simulink model "Dyn_PointMass_r2019b"  (R2022b)
settings: Solver=ode4  StartTime=0.0  StopTime=simInit.TSIM  FixedStep=simInit.dt  MaxStep=simInit.dt  RelTol=1e-3
InitFcn:
  | close all
undefined symbols (not defined in the file): constr, DE2019, DiscIntNeverNeededParam, ENVMT, params, simInit
libraries: simulink x15, simulink_extras x2
(part 1 of 2)
Description:
  | % Copyright 2020 Delft University of Technology
  | %
  | % Licensed under the Apache License, Version 2.0 (the "License");
  | % you may not use this file except in compliance with the License.
  | % You may obtain a copy of the License at
  | %
  | %      http://www.apache.org/licenses/LICENSE-2.0
  | %
  | % Unless required by applicable law or agreed to in writing, software
  | % distributed under the License is distributed on an "AS IS" BASIS,
  | % WITHOUT WARRANTIES OR CONDITIONS OF ANY KIND, either express or implied.
  | % See the License for the specific language governing permissions and
  | % limitations under the License.
settings Model: SimulationMode=accelerator  NumberOfSteps=50  ExtModeTrigDuration=100  Creator=Sebastian  LastModifiedBy=jesse
settings SolverCC: SolverJacobianMethodControl=FullAnalytical  AlgebraicLoopSolver=TrustRegion
settings DataIOCC: InitialState=testPoint  SaveFormat=Structure  SignalLogging=off  DSMLogging=off  SaveTime=off  ReturnWorkspaceOutputs=off  StateSaveName=tmp_raccel_xout  SignalLoggingName=logged_signals  LoggingFileName=log
settings OptimizationCC: BlockReduction=off  EfficientMapNaN2IntZero=off  LifeSpan=inf
settings DebuggingCC: ArtificialAlgebraicLoopMsg=none  SaveWithDisabledLinksMsg=none  SaveWithParameterizedLinksMsg=none  MaskedZcDiagnostic=none  IgnoredZcDiagnostic=none  InheritedTsInSrcMsg=none  TasksWithSamePriorityMsg=none  SigSpecEnsureSampleTimeMsg=none  ParameterPrecisionLossMsg=none  BusObjectLabelMismatch=none  RootOutportRequireBusObject=none  UnknownTsInhSupMsg=none  ModelReferenceDataLoggingMessage=none  ModelReferenceSymbolNameMessage=none  InitInArrayFormatMsg=none  SFUnusedDataAndEventsDiag=none  SFUnexpectedBacktrackingDiag=none  SFInvalidInputDataAccessInChartInitDiag=none  SFNoUnconditionalDefaultTransitionDiag=none  SFTransitionOutsideNaturalParentDiag=none  SFUnreachableExecutionPathDiag=none  SFUndirectedBroadcastEventsDiag=none  SFTransitionActionBeforeConditionDiag=none  SFTemporalDelaySmallerThanSampleTimeDiag=none  SFSelfTransitionDiag=none  SFExecutionAtInitializationDiag=none  SFMachineParentedDataDiag=none  UnitsInconsistencyMsg=none  ArithmeticOperatorsInVariantConditions=warning
settings HardwareCC: ProdBitPerLong=64  ProdLongLongMode=on  ProdHWDeviceType=Custom Processor->Custom Processor  TargetBitPerPointer=64  TargetBitPerSizeT=64  TargetBitPerPtrDiffT=64  TargetLargestAtomicFloat=Float  TargetLongLongMode=on  TargetIntDivRoundTo=Zero  TargetEndianess=LittleEndian  TargetWordSize=64  TargetHWDeviceType=Custom Processor->MATLAB Host Computer
settings ModelReferenceCC: EnableRefExpFcnMdlSchedulingChecks=on  PropagateSignalLabelsOutOfModel=off
settings SFSimCC: SimUseLocalCustomCode=off  CustomCodeUndefinedFunction=UseInterfaceOnly
settings CodeAppCC: MaxIdLength=128
settings GRTTargetCC: TargetLangStandard=C89/C90 (ANSI)  CombineOutputUpdateFcns=off  GRTInterface=on
settings ConfigComp: CovMetricSettings=dw  CovSaveCumulativeToWorkspaceVar=on  CovSaveSingleToWorkspaceVar=on  CovExternalEMLEnable=off
settings SimscapeCC: SimscapeNormalizeSystem=off
settings ConfigurationSet: Description=SimMechanics 2G

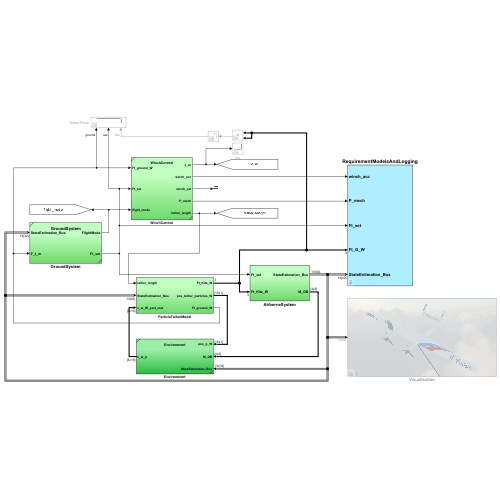
[thumbnail: Simulink's stored preview of the top-level diagram]
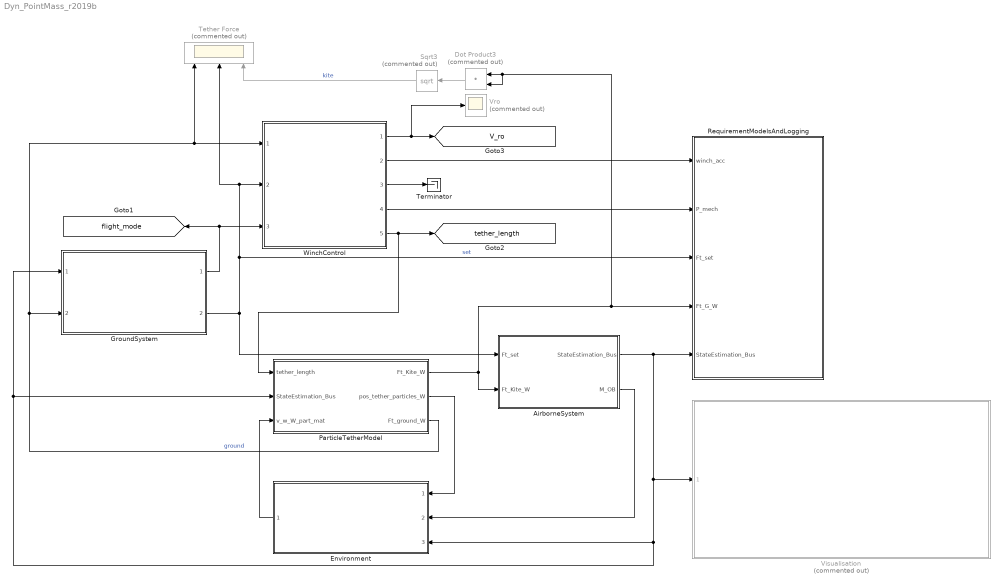
== system Dyn_PointMass_r2019b ==
  AirborneSystem : Subsystem
  Dot Product3 : DotProduct  Commented=on  OutDataTypeStr=Inherit: Inherit via internal rule
  Environment : Subsystem  ReferencedSubsystem=Environment
  GroundSystem : Subsystem  ReferencedSubsystem=GroundSystem
  ParticleTetherModel : Subsystem
  RequirementModelsAndLogging : Subsystem  mask{log_sample_time=0.2}
  Sqrt3 : Sqrt  Commented=on
  Terminator : Terminator
  Tether Force : Scope  Commented=on  NumInputPorts=3
  Visualisation : Subsystem  Commented=on  ReferencedSubsystem=Visualisation  sample_time_vis=1
  Vro : Scope  Commented=on
  WinchControl : Subsystem  ReferencedSubsystem=WinchControl
  tag scope: V_ro=global, flight_mode=global, tether_length=global
  wires:
  GroundSystem/1 -> [flight_mode], WinchControl/3
  GroundSystem/2 -> AirborneSystem/1(Ft_set), RequirementModelsAndLogging/3(Ft_set), Tether Force/2, WinchControl/2  "set"
  AirborneSystem/2(M_OB) -> Environment/2
  AirborneSystem/1(StateEstimation_Bus) -> RequirementModelsAndLogging/5(StateEstimation_Bus), Visualisation/1, GroundSystem/1, ParticleTetherModel/2(StateEstimation_Bus), Environment/3
  ParticleTetherModel/2(pos_tether_particles_W) -> Environment/1
  Environment/1 -> ParticleTetherModel/3(v_w_W_part_mat)
  WinchControl/1 -> Vro/1, [V_ro]
  ParticleTetherModel/3(Ft_ground_W) -> WinchControl/1, Tether Force/1, GroundSystem/2  "ground"
  WinchControl/3 -> Terminator/1
  WinchControl/2 -> RequirementModelsAndLogging/1(winch_acc)
  WinchControl/4 -> RequirementModelsAndLogging/2(P_mech)
  WinchControl/5 -> [tether_length], ParticleTetherModel/1(tether_length)
  Sqrt3/1 -> Tether Force/3  "kite"
  Dot Product3/1 -> Sqrt3/1
  ParticleTetherModel/1(Ft_Kite_W) -> Dot Product3/2, Dot Product3/1, RequirementModelsAndLogging/4(Ft_G_W), AirborneSystem/2(Ft_Kite_W)

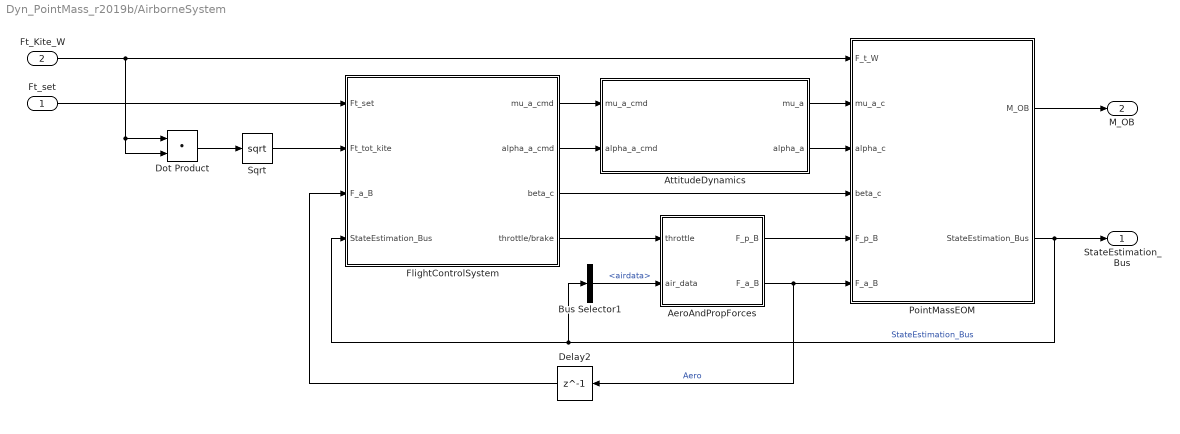
== system Dyn_PointMass_r2019b/AirborneSystem ==
  Ft_set : Inport
  Ft_Kite_W : Inport  Port=2
  AeroAndPropForces : Subsystem
  AttitudeDynamics : Subsystem
  Bus Selector1 : BusSelector  OutputSignals=airdata
  Delay2 : Delay  DelayLength=1  InitialCondition=[0;0;DE2019.mass*ENVMT.g]
  Dot Product : DotProduct  OutDataTypeStr=Inherit: Inherit via internal rule
  FlightControlSystem : Subsystem
  PointMassEOM : Subsystem
  Sqrt : Sqrt
  StateEstimation_Bus : Outport  VectorParamsAs1DForOutWhenUnconnected=off
  M_OB : Outport  Port=2  VectorParamsAs1DForOutWhenUnconnected=off
  wires:
  PointMassEOM/2(StateEstimation_Bus) -> FlightControlSystem/4(StateEstimation_Bus), Bus Selector1/1, StateEstimation_Bus/1  "StateEstimation_Bus"
  PointMassEOM/1(M_OB) -> M_OB/1
  Ft_Kite_W/1 -> PointMassEOM/1(F_t_W), Dot Product/2, Dot Product/1
  Dot Product/1 -> Sqrt/1
  Ft_set/1 -> FlightControlSystem/1(Ft_set)
  Sqrt/1 -> FlightControlSystem/2(Ft_tot_kite)
  FlightControlSystem/4(throttle/brake) -> AeroAndPropForces/1(throttle)
  AeroAndPropForces/1(F_p_B) -> PointMassEOM/5(F_p_B)
  Bus Selector1/1 -> AeroAndPropForces/2(air_data)  "<airdata>"
  AeroAndPropForces/2(F_a_B) -> Delay2/1, PointMassEOM/6(F_a_B)  "Aero"
  AttitudeDynamics/1(mu_a) -> PointMassEOM/2(mu_a_c)
  AttitudeDynamics/2(alpha_a) -> PointMassEOM/3(alpha_c)
  FlightControlSystem/1(mu_a_cmd) -> AttitudeDynamics/1(mu_a_cmd)
  FlightControlSystem/2(alpha_a_cmd) -> AttitudeDynamics/2(alpha_a_cmd)
  FlightControlSystem/3(beta_c) -> PointMassEOM/4(beta_c)
  Delay2/1 -> FlightControlSystem/3(F_a_B)

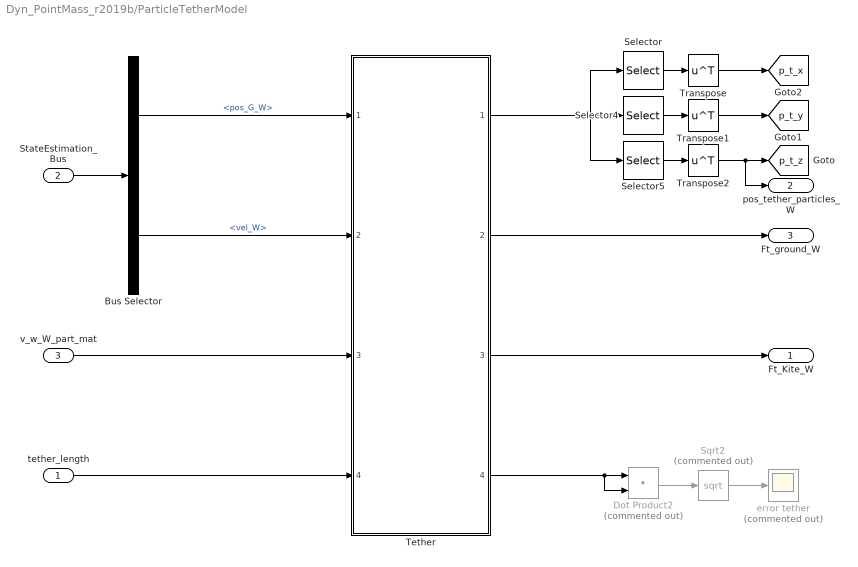
== system Dyn_PointMass_r2019b/ParticleTetherModel ==
  tether_length : Inport
  StateEstimation_Bus : Inport  Port=2
  v_w_W_part_mat : Inport  Port=3
  Bus Selector : BusSelector  OutputSignals=pos_G_W,vel_W
  Dot Product2 : DotProduct  Commented=on  OutDataTypeStr=Inherit: Inherit via internal rule
  Selector : Selector  NumberOfDimensions=2  InputPortWidth=3  IndexOptions=Index vector (dialog),Select all  Indices=1,1  OutputSizes=1,1
  Selector4 : Selector  NumberOfDimensions=2  InputPortWidth=3  IndexOptions=Index vector (dialog),Select all  Indices=2,1  OutputSizes=1,1
  Selector5 : Selector  NumberOfDimensions=2  InputPortWidth=3  IndexOptions=Index vector (dialog),Select all  Indices=3,1  OutputSizes=1,1
  Sqrt2 : Sqrt  Commented=on
  Tether : Subsystem  ReferencedSubsystem=Tether_dynamics_R2019B
  Transpose : Math  Operator=transpose
  Transpose1 : Math  Operator=transpose
  Transpose2 : Math  Operator=transpose
  error tether : Scope  Commented=on
  Ft_Kite_W : Outport  VectorParamsAs1DForOutWhenUnconnected=off
  pos_tether_particles_W : Outport  Port=2  VectorParamsAs1DForOutWhenUnconnected=off
  Ft_ground_W : Outport  Port=3  VectorParamsAs1DForOutWhenUnconnected=off
  tag scope: p_t_x=global, p_t_y=global, p_t_z=global
  wires:
  v_w_W_part_mat/1 -> Tether/3
  StateEstimation_Bus/1 -> Bus Selector/1
  Bus Selector/1 -> Tether/1  "<pos_G_W>"
  Bus Selector/2 -> Tether/2  "<vel_W>"
  Selector4/1 -> Transpose1/1
  Selector5/1 -> Transpose2/1
  Selector/1 -> Transpose/1
  Transpose/1 -> [p_t_x]
  Transpose1/1 -> [p_t_y]
  Transpose2/1 -> pos_tether_particles_W/1, [p_t_z]
  Tether/4 -> Dot Product2/2, Dot Product2/1
  Tether/1 -> Selector/1, Selector5/1, Selector4/1
  Dot Product2/1 -> Sqrt2/1
  Sqrt2/1 -> error tether/1
  Tether/2 -> Ft_ground_W/1
  Tether/3 -> Ft_Kite_W/1
  tether_length/1 -> Tether/4

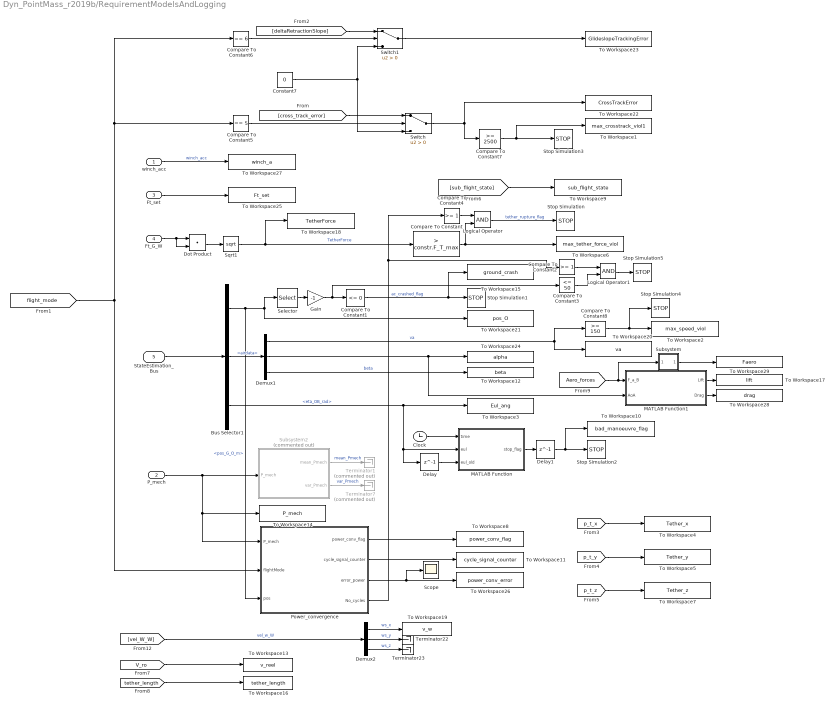
== system Dyn_PointMass_r2019b/RequirementModelsAndLogging ==
  winch_acc : Inport
  P_mech : Inport  Port=2
  Ft_set : Inport  Port=3
  Ft_G_W : Inport  Port=4
  StateEstimation_Bus : Inport  Port=5
  Bus Selector1 : BusSelector  OutputSignals=pos_G_O_m,airdata,eta_OB_rad
  Clock : Clock
  Compare To Constant : simulink/Logic and Bit Operations/Compare To Constant  relop=>  const=constr.F_T_max  OutDataTypeStr=boolean
  Compare To Constant1 : simulink/Logic and Bit Operations/Compare To Constant  relop=<=  const=0  OutDataTypeStr=boolean
  Compare To Constant2 : simulink/Logic and Bit Operations/Compare To Constant  relop=>=  const=1  OutDataTypeStr=boolean
  Compare To Constant3 : simulink/Logic and Bit Operations/Compare To Constant  relop=<=  const=50  OutDataTypeStr=boolean
  Compare To Constant4 : simulink/Logic and Bit Operations/Compare To Constant  relop=>=  const=1  OutDataTypeStr=boolean
  Compare To Constant5 : simulink/Logic and Bit Operations/Compare To Constant  relop===  const=5  OutDataTypeStr=boolean
  Compare To Constant6 : simulink/Logic and Bit Operations/Compare To Constant  relop===  const=6  OutDataTypeStr=boolean
  Compare To Constant7 : simulink/Logic and Bit Operations/Compare To Constant  relop=>=  const=2500  OutDataTypeStr=boolean
  Compare To Constant8 : simulink/Logic and Bit Operations/Compare To Constant  relop=>=  const=150  OutDataTypeStr=boolean
  Constant7 : Constant  Value=0
  Delay : Delay  DelayLength=1  InitialCondition=zeros(3,1)
  Delay1 : Delay  DelayLength=1
  Demux1 : Demux  Outputs=3
  Demux2 : Demux  Outputs=3
  Dot Product : DotProduct  OutDataTypeStr=Inherit: Inherit via internal rule
  Gain : Gain  Gain=-1
  Logical Operator : Logic  AllPortsSameDT=off  OutDataTypeStr=boolean
  Logical Operator1 : Logic  AllPortsSameDT=off  OutDataTypeStr=boolean
  MATLAB Function : MATLAB Function  TreatAsAtomicUnit=on
  MATLAB Function1 : MATLAB Function  TreatAsAtomicUnit=on
  Power_convergence : Subsystem  mask{sample_time=simInit.Ts_power_conv_check, threshold=130000, min_cycles=3, pos_threshold=400}
      mask prompts: threshold "start_threshold"; min_cycles "minimum_cycles"; pos_threshold "maximum position distance"
  Scope : Scope
  Selector : Selector  InputPortWidth=3  IndexOptions=Index vector (dialog)  Indices=3  OutputSizes=1
  Sqrt1 : Sqrt
  Stop Simulation{,1..5} (6 alike) : Stop
  Subsystem : Subsystem
      mask Display: disp('norm()')
  Subsystem2 : Subsystem  Commented=on
  Switch : Switch  Criteria=u2 > Threshold  SaturateOnIntegerOverflow=off  InputSameDT=off
  Switch1 : Switch  Criteria=u2 > Threshold  SaturateOnIntegerOverflow=off  InputSameDT=off
  Terminator1 : Terminator  Commented=on
  Terminator22 : Terminator
  Terminator23 : Terminator
  Terminator7 : Terminator  Commented=on
  To Workspace1 : ToWorkspace  VariableName=max_crosstrack_viol1  SampleTime=-1
      settings: MaxDataPoints=1
  To Workspace10 : ToWorkspace  VariableName=bad_manoeuvre_flag  SampleTime=-1
      settings: MaxDataPoints=1
  To Workspace11 : ToWorkspace  VariableName=cycle_signal_counter  SaveFormat=Timeseries  SampleTime=-1
      settings: MaxDataPoints=1  Save2DSignal=2-D array (concatenate along first dimension)
  To Workspace12 : ToWorkspace  VariableName=beta  SaveFormat=Timeseries  SampleTime=simInit.AttLoggingTs
      settings: Save2DSignal=2-D array (concatenate along first dimension)
  To Workspace13 : ToWorkspace  VariableName=v_reel  SaveFormat=Timeseries  SampleTime=simInit.PLoggingTs
  To Workspace14 : ToWorkspace  VariableName=P_mech  SaveFormat=Timeseries  SampleTime=simInit.PLoggingTs
  To Workspace15 : ToWorkspace  VariableName=ground_crash  SampleTime=-1
      settings: MaxDataPoints=1
  To Workspace16 : ToWorkspace  VariableName=tether_length  SaveFormat=Timeseries  SampleTime=simInit.AttLoggingTs
  To Workspace17 : ToWorkspace  VariableName=lift  SaveFormat=Timeseries  SampleTime=simInit.AttLoggingTs
      settings: Save2DSignal=2-D array (concatenate along first dimension)
  To Workspace18 : ToWorkspace  VariableName=TetherForce  SaveFormat=Timeseries  SampleTime=simInit.FtLoggingTs
  To Workspace19 : ToWorkspace  VariableName=v_w  SaveFormat=Timeseries  SampleTime=simInit.PLoggingTs
  To Workspace2 : ToWorkspace  VariableName=max_speed_viol  SampleTime=-1
      settings: MaxDataPoints=1
  To Workspace20 : ToWorkspace  VariableName=va  SaveFormat=Timeseries  SampleTime=simInit.AttLoggingTs
      settings: Save2DSignal=2-D array (concatenate along first dimension)
  To Workspace21 : ToWorkspace  VariableName=pos_O  SaveFormat=Timeseries  SampleTime=simInit.PLoggingTs
      settings: Save2DSignal=2-D array (concatenate along first dimension)
  To Workspace22 : ToWorkspace  VariableName=CrossTrackError  SaveFormat=Timeseries  SampleTime=simInit.CteLoggingTs
      settings: Save2DSignal=2-D array (concatenate along first dimension)
  To Workspace23 : ToWorkspace  VariableName=GlideslopeTrackingError  SaveFormat=Timeseries  SampleTime=simInit.GSLoggingTs
      settings: Save2DSignal=2-D array (concatenate along first dimension)
  To Workspace24 : ToWorkspace  VariableName=alpha  SaveFormat=Timeseries  SampleTime=simInit.AttLoggingTs
      settings: Save2DSignal=2-D array (concatenate along first dimension)
  To Workspace25 : ToWorkspace  VariableName=Ft_set  SaveFormat=Timeseries  SampleTime=simInit.FtLoggingTs
  To Workspace26 : ToWorkspace  VariableName=power_conv_error  SaveFormat=Timeseries  SampleTime=-1
      settings: Save2DSignal=2-D array (concatenate along first dimension)
  To Workspace27 : ToWorkspace  VariableName=winch_a  SaveFormat=Timeseries  SampleTime=simInit.PLoggingTs
  To Workspace28 : ToWorkspace  VariableName=drag  SaveFormat=Timeseries  SampleTime=simInit.AttLoggingTs
      settings: Save2DSignal=2-D array (concatenate along first dimension)
  To Workspace29 : ToWorkspace  VariableName=Faero  SaveFormat=Timeseries  SampleTime=simInit.AttLoggingTs
      settings: Save2DSignal=2-D array (concatenate along first dimension)
  To Workspace3 : ToWorkspace  VariableName=Eul_ang  SaveFormat=Timeseries  SampleTime=simInit.PLoggingTs
      settings: Save2DSignal=2-D array (concatenate along first dimension)
  To Workspace4 : ToWorkspace  VariableName=Tether_x  SaveFormat=Timeseries  SampleTime=simInit.PLoggingTs
      settings: Save2DSignal=2-D array (concatenate along first dimension)
  To Workspace5 : ToWorkspace  VariableName=Tether_y  SaveFormat=Timeseries  SampleTime=simInit.PLoggingTs
      settings: Save2DSignal=2-D array (concatenate along first dimension)
  To Workspace6 : ToWorkspace  VariableName=max_tether_force_viol  SampleTime=-1
      settings: MaxDataPoints=1
  To Workspace7 : ToWorkspace  VariableName=Tether_z  SaveFormat=Timeseries  SampleTime=simInit.PLoggingTs
      settings: Save2DSignal=2-D array (concatenate along first dimension)
  To Workspace8 : ToWorkspace  VariableName=power_conv_flag  SampleTime=-1
      settings: MaxDataPoints=1
  To Workspace9 : ToWorkspace  VariableName=sub_flight_state  SaveFormat=Timeseries  SampleTime=simInit.FtLoggingTs
  wires:
  Bus Selector1/1 -> Power_convergence/3(pos), Selector/1, To Workspace21/1  "<pos_G_O_m>"
  Gain/1 -> Compare To Constant3/1, Compare To Constant1/1
  Compare To Constant1/1 -> To Workspace15/1, Stop Simulation1/1  "ac_crashed_flag"
  Selector/1 -> Gain/1
  winch_acc/1 -> To Workspace27/1  "winch_acc"
  Logical Operator/1 -> Stop Simulation/1  "tether_rupture_flag"
  Sqrt1/1 -> To Workspace18/1, Compare To Constant/1  "TetherForce"
  StateEstimation_Bus/1 -> Bus Selector1/1
  Power_convergence/1(power_conv_flag) -> To Workspace8/1
  Power_convergence/2(cycle_signal_counter) -> To Workspace11/1
  [vel_W_W] -> Demux2/1  "vel_w_W"
  Bus Selector1/2 -> Demux1/1  "<airdata>"
  Switch/1 -> To Workspace22/1, Compare To Constant7/1
  Subsystem2/1(mean_Pmech) -> Terminator1/1  "mean_Pmech"
  Subsystem2/2(var_Pmech) -> Terminator7/1  "var_Pmech"
  Demux1/1 -> To Workspace20/1, Compare To Constant8/1  "va"
  Demux1/3 -> To Workspace12/1  "beta"
  Demux2/3 -> Terminator23/1  "ws_z"
  Demux2/2 -> Terminator22/1  "ws_y"
  Demux2/1 -> To Workspace19/1  "ws_x"
  Ft_G_W/1 -> Dot Product/2, Dot Product/1
  Dot Product/1 -> Sqrt1/1
  Clock/1 -> MATLAB Function/1(time)
  Compare To Constant4/1 -> Logical Operator/1
  Compare To Constant/1 -> Logical Operator/2, To Workspace6/1
  [flight_mode] -> Compare To Constant6/1, Compare To Constant5/1, Power_convergence/2(flightMode)
  P_mech/1 -> Power_convergence/1(P_mech), To Workspace14/1, Subsystem2/1(P_mech)
  Compare To Constant5/1 -> Switch/2
  [cross_track_error] -> Switch/1
  Switch1/1 -> To Workspace23/1
  [deltaRetractionSlope] -> Switch1/1
  Compare To Constant6/1 -> Switch1/2
  Constant7/1 -> Switch1/3, Switch/3
  Ft_set/1 -> To Workspace25/1
  Power_convergence/3(error_power) -> Scope/1, To Workspace26/1
  Compare To Constant7/1 -> Stop Simulation3/1, To Workspace1/1
  Compare To Constant8/1 -> To Workspace2/1, Stop Simulation4/1
  Bus Selector1/3 -> Delay/1, MATLAB Function/2(eul), To Workspace3/1  "<eta_OB_rad>"
  [p_t_y] -> To Workspace5/1
  [p_t_x] -> To Workspace4/1
  [p_t_z] -> To Workspace7/1
  [sub_flight_state] -> To Workspace9/1
  Delay/1 -> MATLAB Function/3(eul_old)
  MATLAB Function/1(stop_flag) -> Delay1/1
  Delay1/1 -> Stop Simulation2/1, To Workspace10/1
  [V_ro] -> To Workspace13/1
  [tether_length] -> To Workspace16/1
  Power_convergence/4(No_cycles) -> Compare To Constant2/1, Compare To Constant4/1
  Compare To Constant2/1 -> Logical Operator1/1
  Compare To Constant3/1 -> Logical Operator1/2
  Logical Operator1/1 -> Stop Simulation5/1
  MATLAB Function1/1(Lift) -> To Workspace17/1
  [Aero_forces] -> Subsystem/1(In1), MATLAB Function1/1(F_a_B)
  MATLAB Function1/2(Drag) -> To Workspace28/1
  Demux1/2 -> MATLAB Function1/2(AoA), To Workspace24/1
  Subsystem/1(Out1) -> To Workspace29/1

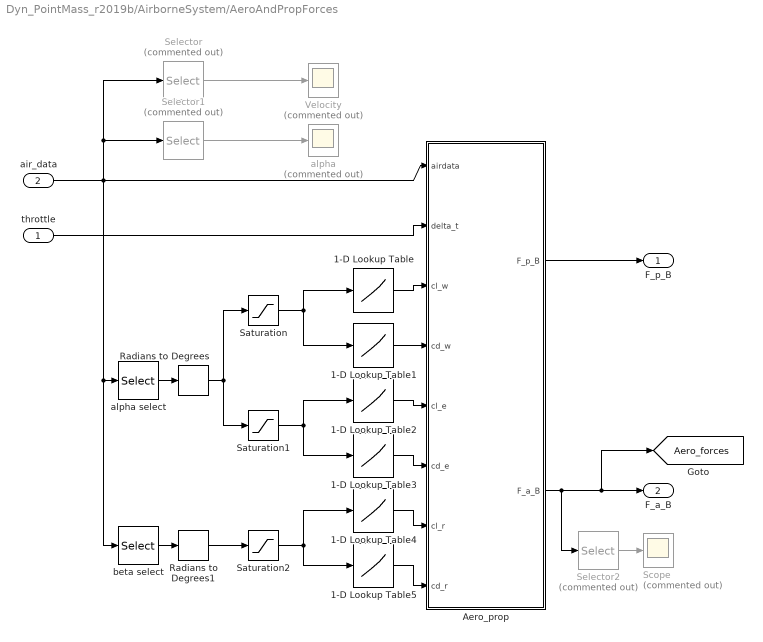
== system Dyn_PointMass_r2019b/AirborneSystem/AeroAndPropForces ==
  throttle : Inport
  air_data : Inport  Port=2
  1-D Lookup Table : Lookup_n-D  NumberOfTableDimensions=1  BreakpointsForDimension1=DE2019.initAircraft.alpha  BreakpointsForDimension2=[1 1]  Table=DE2019.initAircraft.wing_cL_Static'  InternalRulePriority=Speed  RndMeth=Simplest
  1-D Lookup Table1 : Lookup_n-D  NumberOfTableDimensions=1  BreakpointsForDimension1=DE2019.initAircraft.alpha  BreakpointsForDimension2=[1 1]  Table=DE2019.initAircraft.wing_cD_Static'  InternalRulePriority=Speed  RndMeth=Simplest
  1-D Lookup Table2 : Lookup_n-D  NumberOfTableDimensions=1  BreakpointsForDimension1=DE2019.alpha  BreakpointsForDimension2=[1 1]  Table=DE2019.el_cL'  InternalRulePriority=Speed  RndMeth=Simplest
  1-D Lookup Table3 : Lookup_n-D  NumberOfTableDimensions=1  BreakpointsForDimension1=DE2019.alpha  BreakpointsForDimension2=[1 1]  Table=DE2019.el_cD'  InternalRulePriority=Speed  RndMeth=Simplest
  1-D Lookup Table4 : Lookup_n-D  NumberOfTableDimensions=1  BreakpointsForDimension1=DE2019.alpha  BreakpointsForDimension2=[1 1]  Table=DE2019.vs_cL'  InternalRulePriority=Speed  RndMeth=Simplest
  1-D Lookup Table5 : Lookup_n-D  NumberOfTableDimensions=1  BreakpointsForDimension1=DE2019.alpha  BreakpointsForDimension2=[1 1]  Table=DE2019.vs_cD'  InternalRulePriority=Speed  RndMeth=Simplest
  Aero_prop : MATLAB Function  TreatAsAtomicUnit=on
  Radians to Degrees : simulink_extras/Transformations/Radians to Degrees
  Radians to Degrees1 : simulink_extras/Transformations/Radians to Degrees
  Saturation : Saturate  UpperLimit=max(DE2019.initAircraft.alpha)  LowerLimit=min(DE2019.initAircraft.alpha)
  Saturation1 : Saturate  UpperLimit=max(DE2019.alpha)  LowerLimit=min(DE2019.alpha)
  Saturation2 : Saturate  UpperLimit=max(DE2019.alpha)  LowerLimit=min(DE2019.alpha)
  Scope : Scope  Commented=on
  Selector : Selector  Commented=on  InputPortWidth=3  IndexOptions=Index vector (dialog)  Indices=[1]  OutputSizes=1
  Selector1 : Selector  Commented=on  InputPortWidth=3  IndexOptions=Index vector (dialog)  Indices=2  OutputSizes=1
  Selector2 : Selector  Commented=on  InputPortWidth=3  IndexOptions=Index vector (dialog)  Indices=3  OutputSizes=1
  Velocity : Scope  Commented=on
  alpha : Scope  Commented=on
  alpha select : Selector  InputPortWidth=3  IndexOptions=Index vector (dialog)  Indices=2  OutputSizes=1
  beta select : Selector  InputPortWidth=3  IndexOptions=Index vector (dialog)  Indices=3  OutputSizes=1
  F_p_B : Outport  VectorParamsAs1DForOutWhenUnconnected=off
  F_a_B : Outport  Port=2  VectorParamsAs1DForOutWhenUnconnected=off
  tag scope: Aero_forces=global
  wires:
  Aero_prop/1(F_p_B) -> F_p_B/1
  throttle/1 -> Aero_prop/2(delta_t)
  Selector/1 -> Velocity/1
  Selector1/1 -> alpha/1
  1-D Lookup Table/1 -> Aero_prop/3(cl_w)
  1-D Lookup Table1/1 -> Aero_prop/4(cd_w)
  Saturation/1 -> 1-D Lookup Table/1, 1-D Lookup Table1/1
  Saturation1/1 -> 1-D Lookup Table3/1, 1-D Lookup Table2/1
  alpha select/1 -> Radians to Degrees/1
  Radians to Degrees/1 -> Saturation1/1, Saturation/1
  1-D Lookup Table2/1 -> Aero_prop/5(cl_e)
  1-D Lookup Table3/1 -> Aero_prop/6(cd_e)
  1-D Lookup Table4/1 -> Aero_prop/7(cl_r)
  1-D Lookup Table5/1 -> Aero_prop/8(cd_r)
  beta select/1 -> Radians to Degrees1/1
  Radians to Degrees1/1 -> Saturation2/1
  Saturation2/1 -> 1-D Lookup Table4/1, 1-D Lookup Table5/1
  Selector2/1 -> Scope/1
  Aero_prop/2(F_a_B) -> [Aero_forces], F_a_B/1, Selector2/1
  air_data/1 -> Selector/1, Selector1/1, Aero_prop/1(airdata), beta select/1, alpha select/1

== system Dyn_PointMass_r2019b/AirborneSystem/AttitudeDynamics ==
  mu_a_cmd : Inport
  alpha_a_cmd : Inport  Port=2
  Scope : Scope  Commented=on  NumInputPorts=2
  SecondOrderReferenceModel_alpha_a : Subsystem  mask{omega0_max=params.w0_alpha, zeta0=1, y_max=constr.alpha_a_max, y_min=constr.alpha_a_min, yd_max=inf, yd_min=-inf, y2d_max=inf, y2d_min=-inf}
  SecondOrderReferenceModel_mu_a : Subsystem  mask{omega0_max=params.w0_mu, zeta0=1, y_max=constr.mu_a_max, y_min=-constr.mu_a_max, yd_max=inf, yd_min=-inf, y2d_max=inf, y2d_min=-inf}
  mu_a : Outport  VectorParamsAs1DForOutWhenUnconnected=off
  alpha_a : Outport  Port=2  VectorParamsAs1DForOutWhenUnconnected=off
  wires:
  mu_a_cmd/1 -> SecondOrderReferenceModel_mu_a/1(y_cmd)
  SecondOrderReferenceModel_alpha_a/1(y_ref) -> Scope/1, alpha_a/1  "alpha_a"
  alpha_a_cmd/1 -> SecondOrderReferenceModel_alpha_a/1(y_cmd), Scope/2
  SecondOrderReferenceModel_mu_a/1(y_ref) -> mu_a/1  "mu_a"

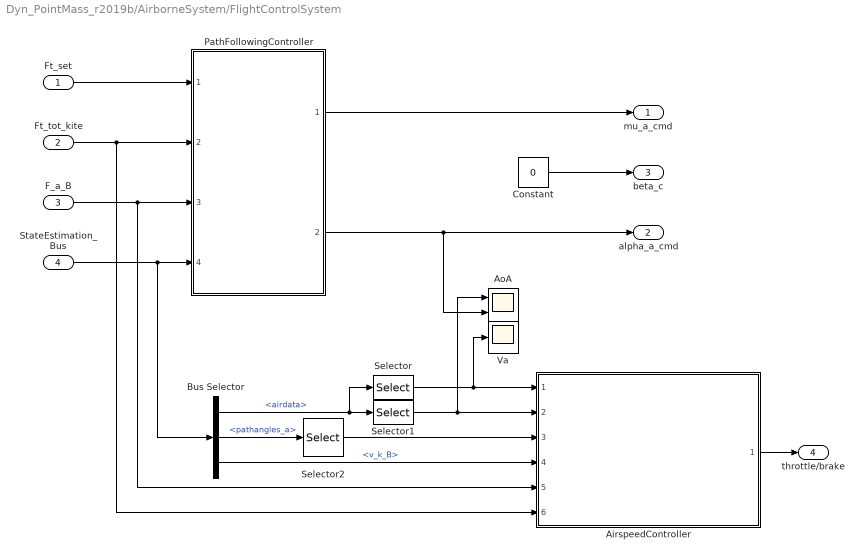
== system Dyn_PointMass_r2019b/AirborneSystem/FlightControlSystem ==
  Ft_set : Inport
  Ft_tot_kite : Inport  Port=2
  F_a_B : Inport  Port=3
  StateEstimation_Bus : Inport  Port=4
  AirspeedController : Subsystem  ReferencedSubsystem=AirspeedController
  AoA : Scope  NumInputPorts=2
  Bus Selector : BusSelector  OutputSignals=airdata,pathangles_a,v_k_B
  Constant : Constant  Value=0
  PathFollowingController : Subsystem  ReferencedSubsystem=PathFollowingController
  Selector : Selector  InputPortWidth=3  IndexOptions=Index vector (dialog)  Indices=1  OutputSizes=1
  Selector1 : Selector  InputPortWidth=3  IndexOptions=Index vector (dialog)  Indices=2  OutputSizes=1
  Selector2 : Selector  InputPortWidth=2  IndexOptions=Index vector (dialog)  Indices=2  OutputSizes=1
  Va : Scope
  mu_a_cmd : Outport  VectorParamsAs1DForOutWhenUnconnected=off
  alpha_a_cmd : Outport  Port=2  VectorParamsAs1DForOutWhenUnconnected=off
  beta_c : Outport  Port=3  VectorParamsAs1DForOutWhenUnconnected=off
  throttle/brake : Outport  Port=4  VectorParamsAs1DForOutWhenUnconnected=off
  wires:
  StateEstimation_Bus/1 -> PathFollowingController/4, Bus Selector/1
  Ft_set/1 -> PathFollowingController/1
  Ft_tot_kite/1 -> PathFollowingController/2, AirspeedController/6
  Bus Selector/1 -> Selector/1, Selector1/1  "<airdata>"
  Selector2/1 -> AirspeedController/3
  Selector/1 -> Va/1, AirspeedController/1
  Selector1/1 -> AoA/1, AirspeedController/2
  F_a_B/1 -> PathFollowingController/3, AirspeedController/5
  Bus Selector/2 -> Selector2/1  "<pathangles_a>"
  AirspeedController/1 -> throttle/brake/1
  Bus Selector/3 -> AirspeedController/4  "<v_k_B>"
  Constant/1 -> beta_c/1
  PathFollowingController/1 -> mu_a_cmd/1
  PathFollowingController/2 -> AoA/2, alpha_a_cmd/1

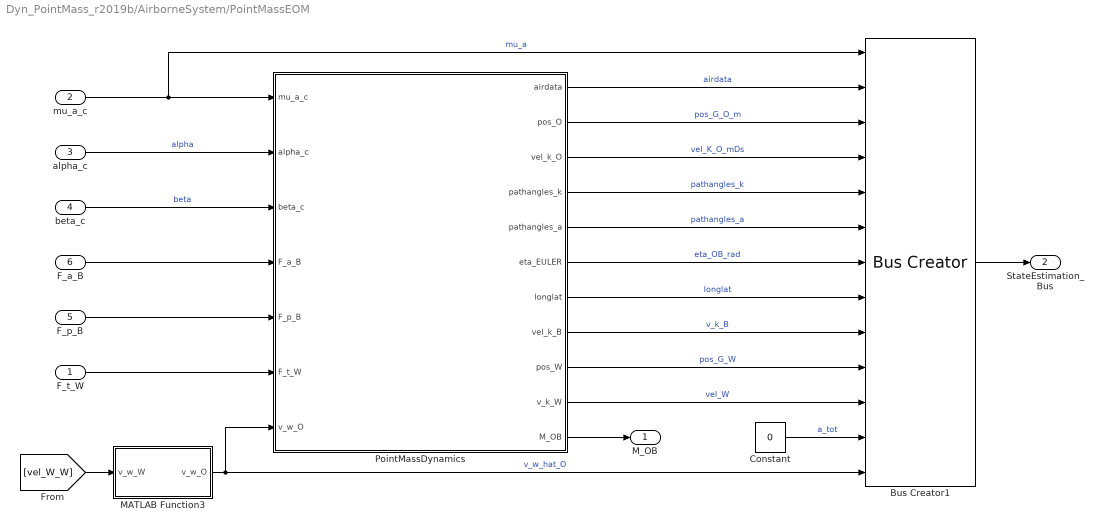
== system Dyn_PointMass_r2019b/AirborneSystem/PointMassEOM ==
  F_t_W : Inport  PortDimensions=[3,1]
  mu_a_c : Inport  Port=2
  alpha_c : Inport  Port=3
  beta_c : Inport  Port=4
  F_p_B : Inport  Port=5  PortDimensions=[3,1]
  F_a_B : Inport  Port=6  PortDimensions=[3,1]
  Bus Creator1 : BusCreator  Inputs=13
  Constant : Constant  Value=0
  MATLAB Function3 : MATLAB Function  TreatAsAtomicUnit=on
  PointMassDynamics : Subsystem
  M_OB : Outport  PortDimensions=[3,3]  VectorParamsAs1DForOutWhenUnconnected=off
  StateEstimation_Bus : Outport  Port=2  VectorParamsAs1DForOutWhenUnconnected=off
  wires:
  mu_a_c/1 -> PointMassDynamics/1(mu_a_c), Bus Creator1/1  "mu_a"
  PointMassDynamics/11(M_OB) -> M_OB/1
  PointMassDynamics/5(pathangles_a) -> Bus Creator1/6  "pathangles_a"
  PointMassDynamics/4(pathangles_k) -> Bus Creator1/5  "pathangles_k"
  PointMassDynamics/6(eta_EULER) -> Bus Creator1/7  "eta_OB_rad"
  PointMassDynamics/7(longlat) -> Bus Creator1/8  "longlat"
  PointMassDynamics/3(vel_k_O) -> Bus Creator1/4  "vel_K_O_mDs"
  Bus Creator1/1 -> StateEstimation_Bus/1
  PointMassDynamics/2(pos_O) -> Bus Creator1/3  "pos_G_O_m"
  MATLAB Function3/1(v_w_O) -> PointMassDynamics/7(v_w_O), Bus Creator1/13  "v_w_hat_O"
  [vel_W_W] -> MATLAB Function3/1(v_w_W)
  PointMassDynamics/9(pos_W) -> Bus Creator1/10  "pos_G_W"
  PointMassDynamics/10(v_k_W) -> Bus Creator1/11  "vel_W"
  PointMassDynamics/1(airdata) -> Bus Creator1/2  "airdata"
  PointMassDynamics/8(vel_k_B) -> Bus Creator1/9  "v_k_B"
  F_p_B/1 -> PointMassDynamics/5(F_p_B)
  F_t_W/1 -> PointMassDynamics/6(F_t_W)
  F_a_B/1 -> PointMassDynamics/4(F_a_B)
  alpha_c/1 -> PointMassDynamics/2(alpha_c)  "alpha"
  beta_c/1 -> PointMassDynamics/3(beta_c)  "beta"
  Constant/1 -> Bus Creator1/12  "a_tot"

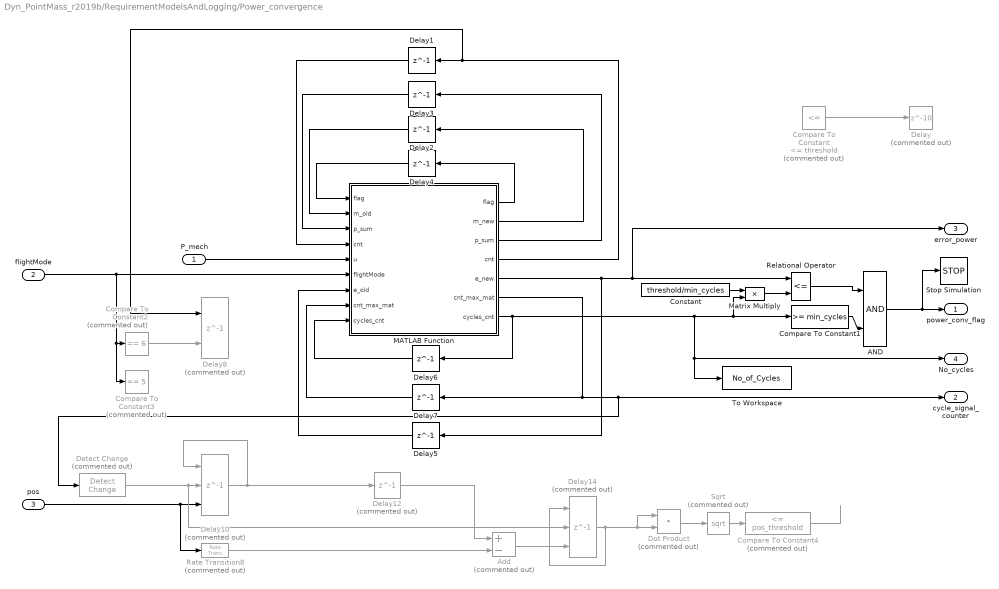
== system Dyn_PointMass_r2019b/RequirementModelsAndLogging/Power_convergence ==
  P_mech : Inport
  flightMode : Inport  Port=2
  pos : Inport  Port=3
  AND : Logic  AllPortsSameDT=off  OutDataTypeStr=boolean
  Add : Sum  Commented=on  Inputs=+-
  Compare To Constant : simulink/Logic and Bit Operations/Compare To Constant  Commented=on  relop=<=  const=threshold  OutDataTypeStr=boolean
  Compare To Constant1 : simulink/Logic and Bit Operations/Compare To Constant  relop=>=  const=min_cycles  OutDataTypeStr=boolean
  Compare To Constant2 : simulink/Logic and Bit Operations/Compare To Constant  Commented=on  relop===  const=6  OutDataTypeStr=boolean
  Compare To Constant3 : simulink/Logic and Bit Operations/Compare To Constant  Commented=on  relop===  const=5  OutDataTypeStr=boolean
  Compare To Constant4 : simulink/Logic and Bit Operations/Compare To Constant  Commented=on  relop=<=  const=pos_threshold  OutDataTypeStr=boolean
  Constant : Constant  Value=threshold/min_cycles
  Delay : Delay  Commented=on  DelayLength=10
  Delay{1..4,6..7} (6 alike) : Delay  DelayLength=1  InitialCondition=0
  Delay10 : Delay  Commented=on  DelayLength=1  InitialConditionSource=Input port  InitialCondition=0  ExternalReset=Rising
      settings: InputPortMap=u0,r5,p4
  Delay12 : Delay  Commented=on  DelayLength=1  InitialCondition=0
  Delay14 : Delay  Commented=on  DelayLength=1  InitialConditionSource=Input port  InitialCondition=0  ExternalReset=Rising
      settings: InputPortMap=u0,r5,p4
  Delay5 : Delay  DelayLength=1  InitialCondition=threshold+1000
  Delay8 : Delay  Commented=on  DelayLength=1  InitialCondition=0  ExternalReset=Rising
      settings: InputPortMap=u0,r5
  Detect Change : simulink/Logic and Bit Operations/Detect Change  Commented=on  vinit=0  OutDataTypeStr=boolean
  Dot Product : DotProduct  Commented=on  OutDataTypeStr=Inherit: Inherit via internal rule
  MATLAB Function : MATLAB Function  TreatAsAtomicUnit=on
  Matrix Multiply : Product
  Rate Transition8 : RateTransition  Commented=on  InitialCondition=[0;0;0]  OutPortSampleTime=sample_time
  Relational Operator : RelationalOperator  Operator=<=  OutDataTypeStr=boolean  RndMeth=Simplest  InputSameDT=off
  Sqrt : Sqrt  Commented=on
  Stop Simulation : Stop
  To Workspace : ToWorkspace  VariableName=No_of_Cycles  SaveFormat=Timeseries  SampleTime=-1
      settings: MaxDataPoints=1
  power_conv_flag : Outport  VectorParamsAs1DForOutWhenUnconnected=off
  cycle_signal_counter : Outport  Port=2  VectorParamsAs1DForOutWhenUnconnected=off
  error_power : Outport  Port=3  VectorParamsAs1DForOutWhenUnconnected=off
  No_cycles : Outport  Port=4
  wires:
  Delay1/1 -> MATLAB Function/4("cnt ")
  P_mech/1 -> MATLAB Function/5(u)
  MATLAB Function/4(cnt) -> Delay8/1, Delay1/1
  Delay2/1 -> MATLAB Function/2(m_old)
  MATLAB Function/1(flag) -> Delay4/1
  Delay4/1 -> MATLAB Function/1("flag ")
  Delay3/1 -> MATLAB Function/3("p_sum ")
  MATLAB Function/3(p_sum) -> Delay3/1
  MATLAB Function/5(e_new) -> Relational Operator/1, error_power/1, Delay5/1
  Delay5/1 -> MATLAB Function/7(e_old)
  AND/1 -> Stop Simulation/1, power_conv_flag/1
  Delay7/1 -> MATLAB Function/8("cnt_max_mat ")
  MATLAB Function/2(m_new) -> Delay2/1
  MATLAB Function/7(cycles_cnt) -> Compare To Constant1/1, Matrix Multiply/2, No_cycles/1, To Workspace/1, Delay6/1
  Delay6/1 -> MATLAB Function/9("cycles_cnt ")
  Relational Operator/1 -> AND/1
  Compare To Constant1/1 -> AND/2
  Compare To Constant2/1 -> Delay8/2
  Compare To Constant/1 -> Delay/1
  Constant/1 -> Matrix Multiply/1
  Matrix Multiply/1 -> Relational Operator/2
  pos/1 -> Rate Transition8/1, Delay10/3
  Sqrt/1 -> Compare To Constant4/1
  Dot Product/1 -> Sqrt/1
  Delay14/1 -> Delay14/1, Dot Product/1, Dot Product/2
  Rate Transition8/1 -> Add/2
  MATLAB Function/6(cnt_max_mat) -> Detect Change/1, cycle_signal_counter/1, Delay7/1
  Delay10/1 -> Delay12/1, Delay10/1
  flightMode/1 -> MATLAB Function/6(flightMode), Compare To Constant3/1, Compare To Constant2/1
  Add/1 -> Delay14/3
  Detect Change/1 -> Delay14/2, Delay10/2
  Compare To Constant4/1 -> ?
  Delay12/1 -> Add/1

== system Dyn_PointMass_r2019b/RequirementModelsAndLogging/Subsystem ==
  In1 : Inport
  Dot Product3 : DotProduct  OutDataTypeStr=Inherit: Inherit via internal rule
  Sqrt1 : Sqrt
  Out1 : Outport
  wires:
  In1/1 -> Dot Product3/1, Dot Product3/2
  Sqrt1/1 -> Out1/1
  Dot Product3/1 -> Sqrt1/1

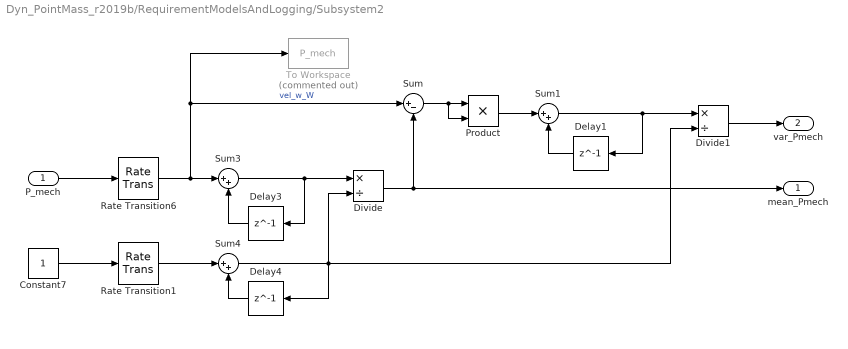
== system Dyn_PointMass_r2019b/RequirementModelsAndLogging/Subsystem2 ==
  P_mech : Inport
  Constant7 : Constant
  Delay1 : Delay  DelayLength=1  SampleTime=0.1
  Delay3 : Delay  DelayLength=1  SampleTime=0.1
  Delay4 : Delay  DelayLength=1  InitialCondition=1  SampleTime=0.1
  Divide : Product  Inputs=*/
  Divide1 : Product  Inputs=*/
  Product : Product
  Rate Transition1 : RateTransition  OutPortSampleTime=0.1
  Rate Transition6 : RateTransition  OutPortSampleTime=0.1
  Sum : Sum  Inputs=|+-
  Sum1 : Sum  Inputs=|++
  Sum3 : Sum  Inputs=|++
  Sum4 : Sum  Inputs=|++
  To Workspace : ToWorkspace  Commented=on  VariableName=P_mech  SampleTime=log_sample_time
  mean_Pmech : Outport  VectorParamsAs1DForOutWhenUnconnected=off
  var_Pmech : Outport  Port=2  VectorParamsAs1DForOutWhenUnconnected=off
  wires:
  P_mech/1 -> Rate Transition6/1
  Delay4/1 -> Sum4/2
  Constant7/1 -> Rate Transition1/1
  Divide/1 -> mean_Pmech/1, Sum/2
  Rate Transition1/1 -> Sum4/1
  Sum3/1 -> Divide/1, Delay3/1
  Sum4/1 -> Divide1/2, Delay4/1, Divide/2
  Delay3/1 -> Sum3/2
  Sum/1 -> Product/2, Product/1
  Product/1 -> Sum1/1
  Delay1/1 -> Sum1/2
  Sum1/1 -> Divide1/1, Delay1/1
  Divide1/1 -> var_Pmech/1
  Rate Transition6/1 -> To Workspace/1, Sum/1, Sum3/1  "vel_w_W"

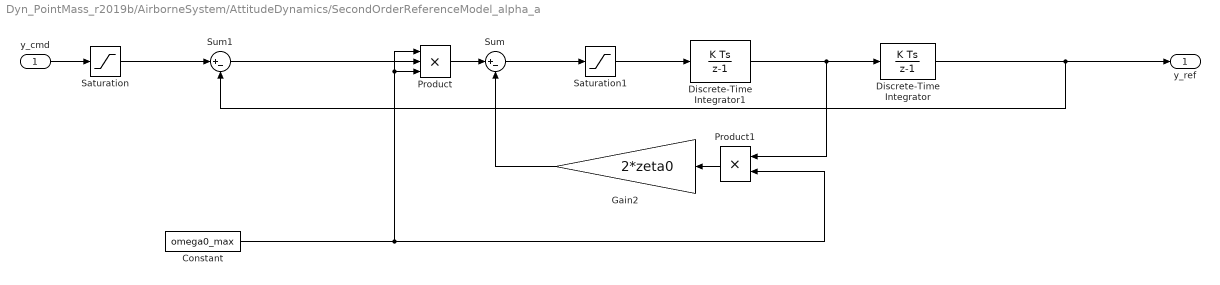
== system Dyn_PointMass_r2019b/AirborneSystem/AttitudeDynamics/SecondOrderReferenceModel_alpha_a ==
  y_cmd : Inport
  Constant : Constant  Value=omega0_max
  Discrete-Time Integrator : DiscreteIntegrator  SampleTime=-1  LimitOutput=on  UpperSaturationLimit=y_max  LowerSaturationLimit=y_min  ICPrevOutput=DiscIntNeverNeededParam  ICPrevScaledInput=DiscIntNeverNeededParam
  Discrete-Time Integrator1 : DiscreteIntegrator  SampleTime=-1  LimitOutput=on  UpperSaturationLimit=yd_max  LowerSaturationLimit=yd_min  ICPrevOutput=DiscIntNeverNeededParam  ICPrevScaledInput=DiscIntNeverNeededParam
  Gain2 : Gain  Gain=2*zeta0
  Product : Product  Inputs=3
  Product1 : Product
  Saturation : Saturate  UpperLimit=y_max  LowerLimit=y_min
  Saturation1 : Saturate  UpperLimit=y2d_max  LowerLimit=y2d_min
  Sum : Sum  Inputs=|+-
  Sum1 : Sum  Inputs=|+-
  y_ref : Outport  VectorParamsAs1DForOutWhenUnconnected=off
  wires:
  Product1/1 -> Gain2/1
  Constant/1 -> Product1/2, Product/3, Product/1
  Product/1 -> Sum/1
  y_cmd/1 -> Saturation/1
  Discrete-Time Integrator1/1 -> Discrete-Time Integrator/1, Product1/1
  Sum/1 -> Saturation1/1
  Gain2/1 -> Sum/2
  Sum1/1 -> Product/2
  Saturation1/1 -> Discrete-Time Integrator1/1
  Saturation/1 -> Sum1/1
  Discrete-Time Integrator/1 -> y_ref/1, Sum1/2

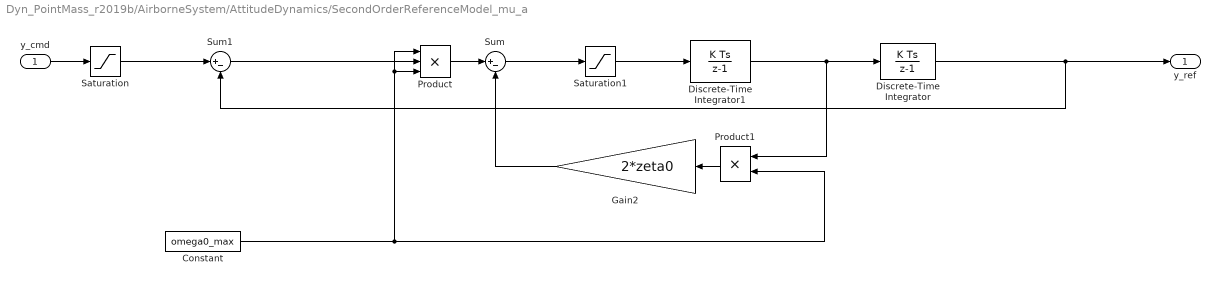
== system Dyn_PointMass_r2019b/AirborneSystem/AttitudeDynamics/SecondOrderReferenceModel_mu_a ==
  y_cmd : Inport
  Constant : Constant  Value=omega0_max
  Discrete-Time Integrator : DiscreteIntegrator  SampleTime=-1  LimitOutput=on  UpperSaturationLimit=y_max  LowerSaturationLimit=y_min  ICPrevOutput=DiscIntNeverNeededParam  ICPrevScaledInput=DiscIntNeverNeededParam
  Discrete-Time Integrator1 : DiscreteIntegrator  SampleTime=-1  LimitOutput=on  UpperSaturationLimit=yd_max  LowerSaturationLimit=yd_min  ICPrevOutput=DiscIntNeverNeededParam  ICPrevScaledInput=DiscIntNeverNeededParam
  Gain2 : Gain  Gain=2*zeta0
  Product : Product  Inputs=3
  Product1 : Product
  Saturation : Saturate  UpperLimit=y_max  LowerLimit=y_min
  Saturation1 : Saturate  UpperLimit=y2d_max  LowerLimit=y2d_min
  Sum : Sum  Inputs=|+-
  Sum1 : Sum  Inputs=|+-
  y_ref : Outport  VectorParamsAs1DForOutWhenUnconnected=off
  wires:
  Product1/1 -> Gain2/1
  Constant/1 -> Product1/2, Product/3, Product/1
  Product/1 -> Sum/1
  y_cmd/1 -> Saturation/1
  Discrete-Time Integrator1/1 -> Discrete-Time Integrator/1, Product1/1
  Sum/1 -> Saturation1/1
  Gain2/1 -> Sum/2
  Sum1/1 -> Product/2
  Saturation1/1 -> Discrete-Time Integrator1/1
  Saturation/1 -> Sum1/1
  Discrete-Time Integrator/1 -> y_ref/1, Sum1/2

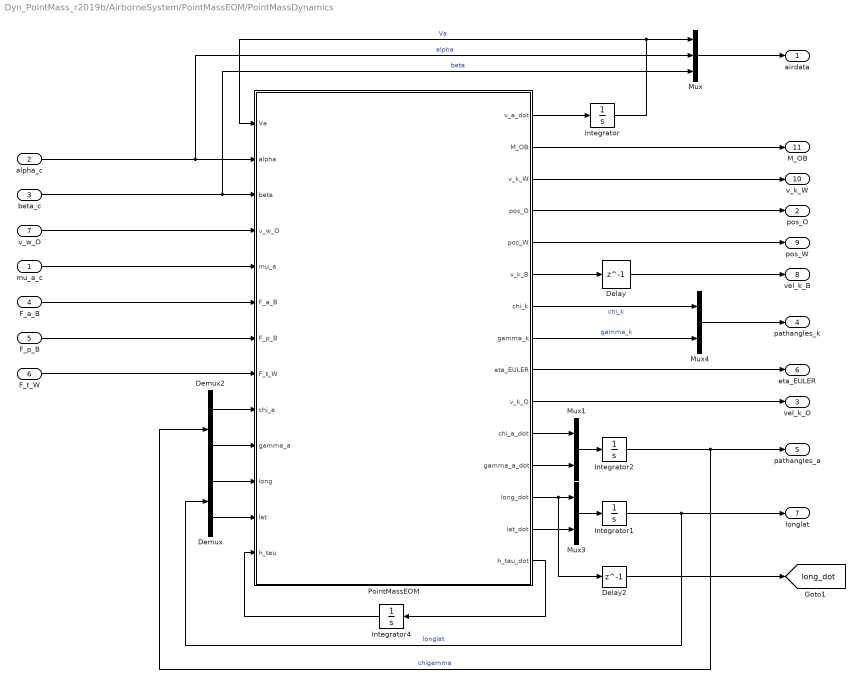
== system Dyn_PointMass_r2019b/AirborneSystem/PointMassEOM/PointMassDynamics ==
  mu_a_c : Inport
  alpha_c : Inport  Port=2
  beta_c : Inport  Port=3
  F_a_B : Inport  Port=4  PortDimensions=[3,1]
  F_p_B : Inport  Port=5  PortDimensions=[3,1]
  F_t_W : Inport  Port=6  PortDimensions=[3,1]
  v_w_O : Inport  Port=7
  Delay : Delay  DelayLength=1  InitialCondition=simInit.vel_B_init
  Delay2 : Delay  DelayLength=1
  Demux : Demux  Outputs=2
  Demux2 : Demux  Outputs=2
  Integrator : Integrator  InitialCondition=simInit.vel_B_init(1)
  Integrator1 : Integrator  InitialCondition=[simInit.long_init;simInit.lat_init]  WrapState=on
  Integrator2 : Integrator  InitialCondition=zeros(2,1)  WrapState=on
  Integrator4 : Integrator  InitialCondition=norm(simInit.pos_O_init)
  Mux : Mux  Inputs=3
  Mux1 : Mux  Inputs=2
  Mux3 : Mux  Inputs=2
  Mux4 : Mux  Inputs=2
  PointMassEOM : MATLAB Function  TreatAsAtomicUnit=on
  airdata : Outport  PortDimensions=3  VectorParamsAs1DForOutWhenUnconnected=off
  pos_O : Outport  Port=2  PortDimensions=[3,1]  VectorParamsAs1DForOutWhenUnconnected=off
  vel_k_O : Outport  Port=3  PortDimensions=[3,1]  VectorParamsAs1DForOutWhenUnconnected=off
  pathangles_k : Outport  Port=4  PortDimensions=2  VectorParamsAs1DForOutWhenUnconnected=off
  pathangles_a : Outport  Port=5  PortDimensions=2  VectorParamsAs1DForOutWhenUnconnected=off
  eta_EULER : Outport  Port=6  PortDimensions=[3,1]  VectorParamsAs1DForOutWhenUnconnected=off
  longlat : Outport  Port=7  PortDimensions=2  VectorParamsAs1DForOutWhenUnconnected=off
  vel_k_B : Outport  Port=8  PortDimensions=[3,1]  VectorParamsAs1DForOutWhenUnconnected=off
  pos_W : Outport  Port=9  PortDimensions=[3,1]  VectorParamsAs1DForOutWhenUnconnected=off
  v_k_W : Outport  Port=10  PortDimensions=[3,1]  VectorParamsAs1DForOutWhenUnconnected=off
  M_OB : Outport  Port=11  PortDimensions=[3,3]  VectorParamsAs1DForOutWhenUnconnected=off
  tag scope: long_dot=global
  wires:
  F_p_B/1 -> PointMassEOM/7(F_p_B)
  mu_a_c/1 -> PointMassEOM/5(mu_a)
  PointMassEOM/7(chi_k) -> Mux4/1  "chi_k"
  F_a_B/1 -> PointMassEOM/6(F_a_B)
  Integrator/1 -> PointMassEOM/1(Va), Mux/1  "Va"
  PointMassEOM/8(gamma_k) -> Mux4/2  "gamma_k"
  PointMassEOM/12(gamma_a_dot) -> Mux1/2
  Integrator4/1 -> PointMassEOM/13(h_tau)
  PointMassEOM/14(lat_dot) -> Mux3/2
  PointMassEOM/11(chi_a_dot) -> Mux1/1
  PointMassEOM/15(h_tau_dot) -> Integrator4/1
  PointMassEOM/1(v_a_dot) -> Integrator/1
  Demux2/2 -> PointMassEOM/10(gamma_a)
  v_w_O/1 -> PointMassEOM/4(v_w_O)
  PointMassEOM/9(eta_EULER) -> eta_EULER/1
  Mux/1 -> airdata/1
  alpha_c/1 -> Mux/2, PointMassEOM/2(alpha)  "alpha"
  beta_c/1 -> Mux/3, PointMassEOM/3(beta)  "beta"
  PointMassEOM/10(v_k_O) -> vel_k_O/1
  PointMassEOM/6(v_k_B) -> Delay/1
  PointMassEOM/5(pos_W) -> pos_W/1
  PointMassEOM/4(pos_O) -> pos_O/1
  Demux2/1 -> PointMassEOM/9(chi_a)
  PointMassEOM/3(v_k_W) -> v_k_W/1
  PointMassEOM/2(M_OB) -> M_OB/1
  PointMassEOM/13(long_dot) -> Mux3/1, Delay2/1
  Mux3/1 -> Integrator1/1
  Delay2/1 -> [long_dot]
  Integrator1/1 -> longlat/1, Demux/1  "longlat"
  Demux/1 -> PointMassEOM/11(long)
  Demux/2 -> PointMassEOM/12(lat)
  Mux1/1 -> Integrator2/1
  Integrator2/1 -> pathangles_a/1, Demux2/1  "chigamma"
  F_t_W/1 -> PointMassEOM/8(F_t_W)
  Delay/1 -> vel_k_B/1
  Mux4/1 -> pathangles_k/1

== matlab function Dyn_PointMass_r2019b/RequirementModelsAndLogging/MATLAB Function1 ==
  data: Lift output; F_a_B input; Drag output; AoA input
% Copyright 2021 Delft University of Technology
%
% Licensed under the Apache License, Version 2.0 (the "License");
% you may not use this file except in compliance with the License.
% You may obtain a copy of the License at
%
%      http://www.apache.org/licenses/LICENSE-2.0
%
% Unless required by applicable law or agreed to in writing, software
% distributed under the License is distributed on an "AS IS" BASIS,
% WITHOUT WARRANTIES OR CONDITIONS OF ANY KIND, either express or implied.
% See the License for the specific language governing permissions and
% limitations under the License.

function [Lift, Drag]  = estimate_drag(F_a_B, AoA)
%estimate_drag - Transform drag from B to A reference frame
%
% Inputs:
%    F_a_B     - Aerodynamic forces in body reference frame
%    AoA       - Angle of Attack
%
% Outputs:
%    Drag    - Drag force
%
% Example: 
%    [Drag] = estimate_drag(F_a_B, AoA)
%
% Author: Sebastian Rapp, Ph.D., Revised by: Dylan Eijkelhof, M.Sc.
% Delft University of Technology
% email address: s.rapp@tudelft.nl
% email address: d.eijkelhof@tudelft.nl
% December 2019; Last revision: 06-October-2020

%-------------	BEGIN CODE	--------------

F_a_A = [cos(AoA), 0, sin(AoA);
    0, 1, 0; 
    -sin(AoA), 0, cos(AoA)] * F_a_B;

Lift = -F_a_A(3);
Drag = -F_a_A(1);

%-------------	 END CODE	--------------

end

== matlab function Dyn_PointMass_r2019b/AirborneSystem/PointMassEOM/MATLAB Function3 ==
  data: v_w_O output; v_w_W input; ENVMT parameter
% Copyright 2020 Delft University of Technology
%
% Licensed under the Apache License, Version 2.0 (the "License");
% you may not use this file except in compliance with the License.
% You may obtain a copy of the License at
%
%      http://www.apache.org/licenses/LICENSE-2.0
%
% Unless required by applicable law or agreed to in writing, software
% distributed under the License is distributed on an "AS IS" BASIS,
% WITHOUT WARRANTIES OR CONDITIONS OF ANY KIND, either express or implied.
% See the License for the specific language governing permissions and
% limitations under the License.

function v_w_O = fcn(v_w_W, ENVMT)



M_OW = [cos(ENVMT.windDirection_rad), sin(ENVMT.windDirection_rad), 0;
        sin(ENVMT.windDirection_rad), -cos(ENVMT.windDirection_rad), 0;
        0, 0, -1];

v_w_O =M_OW*v_w_W;

== matlab function Dyn_PointMass_r2019b/RequirementModelsAndLogging/Power_convergence/MATLAB Function ==
  settings: updateMethod=DISCRETE  sampleTime=simInit.Ts_power_conv_check
  data: flag output; m_new output; p_sum output; cnt output; flag input; m_old input; p_sum input; cnt input; u input; flightMode input; e_new output; e_old input; cnt_max_mat input; cnt_max_mat output; cycles_cnt input; cycles_cnt output
% Copyright 2021 Delft University of Technology
%
% Licensed under the Apache License, Version 2.0 (the "License");
% you may not use this file except in compliance with the License.
% You may obtain a copy of the License at
%
%      http://www.apache.org/licenses/LICENSE-2.0
%
% Unless required by applicable law or agreed to in writing, software
% distributed under the License is distributed on an "AS IS" BASIS,
% WITHOUT WARRANTIES OR CONDITIONS OF ANY KIND, either express or implied.
% See the License for the specific language governing permissions and
% limitations under the License.

function [flag, m_new, p_sum, cnt, e_new, cnt_max_mat,cycles_cnt] = fcn(flag, m_old, p_sum, cnt, u, flightMode, e_old,cnt_max_mat,cycles_cnt)
% function [flag, m_new, p_sum, cnt, e_new, cnt_max_mat,cycles_cnt] = fcn(flag, m_old, p_sum, cnt, u, flightMode, e_old,cnt_max_mat,cycles_cnt, cnt_extra)
%y = [u;old(1:end-1)];
% if cnt > nmax
%     new_mean = mean(y);
%     cnt = 0;
% end
p_sum = p_sum + u;
cnt = cnt + 1;

if flightMode == 5 && flag
    cnt_max_mat = cnt; 
    m_new = p_sum/cnt;
    cnt  = 0;
    cycles_cnt = cycles_cnt + 1;
    p_sum = 0;
    flag = 0;
    e_new = abs( m_new - m_old );
elseif flightMode == 6
%     if cnt_extra == 0 || cycles_cnt == 0
%         cycles_cnt = cycles_cnt + 1;
%     end
    flag = 1;
    m_new = m_old;
    e_new = e_old;
else
    flag = 0;
    m_new = m_old;
    e_new = e_old;
end

% m_new = m_old + (u-old(nmax))/nmax;

== matlab function Dyn_PointMass_r2019b/AirborneSystem/PointMassEOM/PointMassDynamics/PointMassEOM ==
  data: Va input; alpha input; beta input; v_a_dot output; M_OB output; v_k_W output; pos_O output; pos_W output; v_k_B output; chi_k output; gamma_k output; eta_EULER output; v_k_O output; v_w_O input; mu_a input; F_a_B input; F_p_B input; F_t_W input; chi_a input; gamma_a input; long input; lat input; h_tau input; DE2019 parameter; ENVMT parameter; chi_a_dot output; gamma_a_dot output; long_dot output; lat_dot output; h_tau_dot output
% Copyright 2020 Delft University of Technology
%
% Licensed under the Apache License, Version 2.0 (the "License");
% you may not use this file except in compliance with the License.
% You may obtain a copy of the License at
%
%      http://www.apache.org/licenses/LICENSE-2.0
%
% Unless required by applicable law or agreed to in writing, software
% distributed under the License is distributed on an "AS IS" BASIS,
% WITHOUT WARRANTIES OR CONDITIONS OF ANY KIND, either express or implied.
% See the License for the specific language governing permissions and
% limitations under the License.

function [v_a_dot, M_OB, v_k_W, pos_O,pos_W, v_k_B, chi_k, gamma_k,eta_EULER, ...
    v_k_O, chi_a_dot,gamma_a_dot,long_dot,lat_dot,h_tau_dot] = pmEOM(Va, alpha, ...
    beta, v_w_O, mu_a, F_a_B, F_p_B, F_t_W, chi_a, gamma_a, long, lat,h_tau, DE2019, ENVMT)
%pmEOM - Solve adapted equations of motion for a point mass dynamic system
%
% Inputs:
%    Va       - Aircraft velocity component on body x axis
%    alpha    - Aircraft angle of attack
%    beta     - Aircraft side slip angle
%    v_w_O    - Wind velocity at aircraft in inertial reference frame
%    mu_a     - Roll angle aircraft in body reference frame
%    F_a_B    - Aerodynamic forces in body reference frame
%    F_p_B    - Propulsion forces in body reference frame
%    F_t_W    - Tether tension at aircraft in wind reference frame
%    chi_a    - Aerodynamic course heading
%    gamma_a  - Aerodynamic path angle
%    long     - Longtitude, ground station center of earth
%    lat      - Latitude, ground station center of earth
%    h_tau    - Distance from gound station
%    DE2019   - Aircraft parameters in data structure format
%    ENVMT    - Environmental properties
%
% Outputs:
%    v_a_dot        - Aircraft acceleration on body x axis
%    M_OB           - Transformation matrix between inertial and body
%                     reference frames
%    v_k_W          - Kinetic velocity in wind reference frame
%    pos_O          - Aircraft position in inertial reference frame
%    pos_W          - Aircraft position in wind reference frame
%    v_k_B          - Kinetic velocity in body reference frame
%    chi_k          - Kinetic course heading
%    gamma_k        - Kinetic path angle
%    eta_EULER      - Euler angles aircraft
%    v_k_O          - Kinetic velocity in inertial reference frame
%    chi_a_dot      - Time derivative course heading
%    gamma_a_dot    - Time derivative path angle
%    long_dot       - Time derivative longtitude
%    lat_dot        - Time derivative longtitude
%    h_tau_dot      - Time derivative distance from ground station
%
% Example: 
%    [v_a_dot, M_OB, v_k_W, pos_O,pos_W, v_k_B, chi_k, gamma_k,eta_EULER, ...
%     v_k_O, chi_a_dot,gamma_a_dot,long_dot,lat_dot,h_tau_dot] = pmEOM(Va, alpha, ...
%     beta, v_w_O, mu_a, F_a_B, F_p_B, F_t_W, chi_a, gamma_a, long, lat,h_tau, DE2019, ENVMT)
%
% Other m-files required: none
% Subfunctions: none
% MAT-files required: none
%
% Author: Sebastian Rapp, Phd.
% Delft University of Technology
% email address: s.rapp@tudelft.nl  

%------------- BEGIN CODE --------------

%% Pre-allocation of variables for codegen
beta_k= 0;
alpha_k= 0;
chi_k = 0;
gamma_k  = 0;
M_OB = zeros(3); 
eta_EULER = zeros(3,1); 

%% Initiate variables and transformation matrices
M_BA = [cos(alpha), 0, -sin(alpha); 
    0, 1, 0; 
 sin(alpha), -sin(alpha), cos(alpha)];

M_AB = M_BA.';

s_lat = sin(lat); 
s_long = sin(long); 
c_lat = cos(lat); 
c_long = cos(long); 

M_tauW = [-s_lat *c_long, -s_lat *s_long, c_lat;
    -s_long, c_long, 0;
    -c_lat*c_long, -c_lat*s_long, -s_lat ];

xi = ENVMT.windDirection_rad;
M_OW = [cos(xi), sin(xi), 0; 
    sin(xi), -cos(xi), 0; 
    0, 0, -1];
M_WO = M_OW; 

cos_ca = cos(chi_a); 
cos_ga = cos(gamma_a); 
sin_ca = sin(chi_a); 
sin_ga = sin(gamma_a); 

M_AbarO = [cos_ca*cos_ga, sin_ca*cos_ga, -sin_ga; 
    -sin_ca, cos_ca, 0; 
    cos_ca*sin_ga, sin_ca*sin_ga, cos_ga];
M_OAbar = M_AbarO';
M_AbarA = [1,0,0; 
            0, cos(mu_a), -sin(mu_a); 
            0, sin(mu_a), cos(mu_a)];
M_AAbar = M_AbarA';

%%
v_a_O = M_OAbar*[Va;0;0]; 
v_a_B = M_BA*[Va;0;0]; 
v_w_B = M_BA*M_AAbar*M_AbarO*v_w_O;
v_k_B = v_a_B + v_w_B; 
v_k_O = v_a_O + v_w_O; 
v_k_W = M_WO*v_k_O; 
Vk = norm(v_k_B); 

chi_k = atan2( v_k_O(2), v_k_O(1) ); 
gamma_k = -asin( 1/Vk*v_k_O(3) ); 


Ft_Abar = M_AbarO*M_OW*F_t_W;
Fa_Abar = M_AbarA*M_AB*F_a_B; 
Fp_Abar = M_AbarA*M_AB*F_p_B; 
Fg_Abar = M_AbarO*[0;0;DE2019.mass*ENVMT.g];

Ftot_Abar = Ft_Abar + Fg_Abar + Fa_Abar + Fp_Abar; 
x_dot_Abar = 1/DE2019.mass*diag([1,1/(Va*cos_ga),-1/Va]) * Ftot_Abar; 
% states are: Va, chi_a, gamma_a
v_a_dot = x_dot_Abar(1); 
chi_a_dot = x_dot_Abar(2);
gamma_a_dot = x_dot_Abar(3); 

v_k_tau =M_tauW*v_k_W;

long_dot = v_k_tau(2)/( abs(h_tau)*cos(lat));
lat_dot = v_k_tau(1)/abs(h_tau);
h_tau_dot = -v_k_tau(3);

pos_W= [cos(long)*cos(lat); sin(long)*cos(lat); sin(lat)]*h_tau;
pos_O = M_OW*pos_W; 
M_OB = M_OAbar * M_AbarA * M_AB;

%% Calculate euler angles, roll pitch yaw in inertial reference frame
PHI =  atan2( M_OB(3,2), M_OB(3,3) ); 
THETA = -asin( M_OB(3,1) ); 
PSI = atan2( M_OB(2,1), M_OB(1,1) ); 

eta_EULER = [PHI; THETA; PSI];

%------------- END CODE --------------
end
